simulink model "swingup_controller"  (R2015b)
settings: Solver=FixedStepDiscrete  StartTime=0.0  StopTime=tstop  FixedStep=T  RelTol=1e-3
values from neighbouring files (symbols this model uses):
  ABSALPHA_ON = 22.5 + (5)    (= 27.5)    [swingup_setup.m]
  Ad = ss_disc.A    [balance_setup.m]    (also in swingup_setup.m)
  alpha_cal = -(360/4096) * (pi/180)    (= -0.00153398078789)    [balance_setup.m]    (also in swingup_setup.m)
  ALPHAUR_ON = 60    [swingup_setup.m]
  Bd = ss_disc.B    [balance_setup.m]    (also in swingup_setup.m)
  bemf_lim = .25    (= 0.25)    [swingup_setup.m]
  Cd = ss_disc.C    [balance_setup.m]    (also in swingup_setup.m)
  Dd = ss_disc.D    [balance_setup.m]    (also in swingup_setup.m)
  Er = 0.42    [swingup_setup.m]
  eta_g = 0.9    [swingup_setup.m]
  eta_m = 0.69    [swingup_setup.m]
  g = 9.81    [swingup_setup.m]
  Jp = 0.0012    [swingup_setup.m]
  Kg = 70    [swingup_setup.m]
  km = 7.68e-3    (= 0.00768)    [swingup_setup.m]
  kt = 0.00768    [swingup_setup.m]
  Lp = 0.337    [swingup_setup.m]
  Lr = 0.216    [swingup_setup.m]
  Mp = 0.127    [swingup_setup.m]
  Mr = 0.257    [swingup_setup.m]
  mu = 5.5    [swingup_setup.m]
  Rm = 2.6    [swingup_setup.m]
  T = 0.001    [balance_setup.m]    (also in swingup_setup.m)
  theta_cal = -(360/4096) * (pi/180)    (= -0.00153398078789)    [balance_setup.m]    (also in swingup_setup.m)
  theta_HARDLIM = 160/180 * pi    (= 2.79252680319)    [swingup_setup.m]
  umax = 5    [swingup_setup.m]
  umax_LIM = tau/(Mr*Lr)    (= 11.565399581)    [swingup_setup.m]
  Vin_HARDLIM = 5    [swingup_setup.m]
undefined symbols (not defined in the file or in its folder): denV, Discrete, HIL, K_lqr, numV, Time
libraries: simulink x5, quarc_library x4, ctrlSharedLib x1
settings Model: SimulationMode=external  ExtModeTrigType=signal  ExtModeTrigDuration=200000  ExtModeTrigDirection=either  ExtModeTrigLevel=0.500000  Creator=shadar  LastModifiedBy=maxcrisafulli
settings SolverCC: PositivePriorityOrder=on
settings RTWCC: SystemTargetFile=quarc_win64.tlc  TemplateMakefile=quarc_default_tmf  Description=QUARC Win64 Target
settings STFCustomTargetCC: GeneratePreprocessorConditionals=Use local settings  CPPClassGenCompliant=off
settings GRTTargetCC: ParMdlRefBuildCompliant=off  CompOptLevelCompliant=off  CombineOutputUpdateFcns=off  MatFileLogging=off  CPPClassGenCompliant=off  GRTInterface=on  UseToolchainInfoCompliant=off  ExtMode=on  ExtModeMexFile=quarc_comm

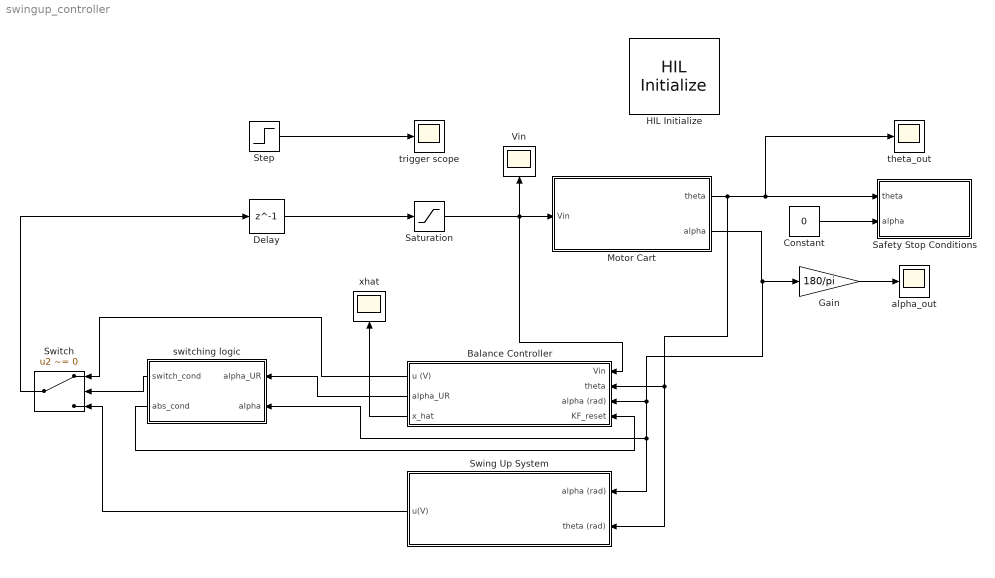
== system swingup_controller ==
  Balance Controller : Subsystem
  Constant : Constant  Value=0
  Delay : Delay  DelayLength=1  InitialCondition=0
  Gain : Gain  Gain=180/pi
  HIL Initialize : quarc_library/Data Acquisition/Generic/Configuration/HIL Initialize  object_name=HIL-1  board_type=q4  board_number=0  board_options=""  exclusive=off  active=on  hardware_clocks=[0:1]  clock_modes=[0 0]  initial_clock_frequencies=[]  set_clock_params_at_start=on  set_clock_params_at_switch_in=off  set_clock_frequencies_at_start=off  set_clock_frequencies_at_switch_in=off  analog_input_channels=[0:3]  analog_input_configurations=[]  analog_input_maximums=10  analog_input_minimums=-10  set_analog_input_params_at_start=off  set_analog_input_params_at_switch_in=off  analog_output_channels=[0:3]  analog_output_maximums=[10]  analog_output_minimums=[-10]  initial_analog_outputs=[0]  final_analog_outputs=[0]  watchdog_analog_outputs=0  set_analog_output_params_at_start=on  set_analog_output_params_at_switch_in=off  set_analog_outputs_at_start=on  set_analog_outputs_at_switch_in=off  set_analog_outputs_at_terminate=on  set_analog_outputs_at_switch_out=off  set_analog_outputs_on_watchdog=off  digital_input_channels=[]  digital_output_channels=[]  digital_output_configuration=[]  initial_digital_outputs=[1]  final_digital_outputs=[1]  watchdog_digital_outputs=[2]  set_digital_output_params_at_start=off  set_digital_output_params_at_switch_in=off  set_digital_outputs_at_start=on  set_digital_outputs_at_switch_in=off  set_digital_outputs_at_terminate=on  set_digital_outputs_at_switch_out=off  set_digital_outputs_on_watchdog=off  encoder_channels=[0:3]  quadrature=[4]  encoder_filter_frequency=(1/60e-9)/1  initial_encoder_counts=[0]  set_encoder_params_at_start=on  set_encoder_params_at_switch_in=off  set_encoder_counts_at_start=on  set_encoder_counts_at_switch_in=off  pwm_channels=[]  pwm_modes=[0]  pwm_frequency=(1/60e-9)/1024  pwm_configuration=[]  pwm_alignment=[]  pwm_polarity=[]  pwm_leading_deadband=[]  pwm_trailing_deadband=[]  initial_pwm_outputs=[0]  final_pwm_outputs=[0]  watchdog_pwm_outputs=[]  set_pwm_params_at_start=on  set_pwm_params_at_switch_in=off  set_pwm_outputs_at_start=on  set_pwm_outputs_at_switch_in=off  set_pwm_outputs_at_terminate=on  set_pwm_outputs_at_switch_out=off  set_pwm_outputs_on_watchdog=off  other_output_channels=[]  initial_other_outputs=[]  final_other_outputs=[]  watchdog_other_outputs=[]  set_other_outputs_at_start=off  set_other_outputs_at_switch_in=off  set_other_outputs_at_terminate=off  set_other_outputs_at_switch_out=off  set_other_outputs_on_watchdog=off
  "Motor Cart " : Subsystem
  Safety Stop Conditions : Subsystem
  Saturation : Saturate  UpperLimit=Vin_HARDLIM  LowerLimit=-Vin_HARDLIM
  Step : Step  Time=0.001  SampleTime=0
  Swing Up System : Subsystem
  Switch : Switch  Criteria=u2 ~= 0  Threshold=15/180 * pi
  Vin : Scope
  "alpha_out " : Scope
  switching logic : Subsystem
  theta_out : Scope
  trigger scope : Scope
  xhat : Scope
  wires:
  Step/1 -> trigger scope/1
  "Motor Cart "/1(theta) -> theta_out/1, Safety Stop Conditions/1(theta), Swing Up System/2(theta (rad)), Balance Controller/2(theta)
  "Motor Cart "/2(alpha) -> Swing Up System/1(alpha (rad)), switching logic/2(alpha), Balance Controller/3(alpha (rad)), Gain/1
  Saturation/1 -> Balance Controller/1(Vin), "Motor Cart "/1(Vin), Vin/1
  Delay/1 -> Saturation/1
  Constant/1 -> Safety Stop Conditions/2(alpha)
  Swing Up System/1(u(V)) -> Switch/3
  Switch/1 -> Delay/1
  Gain/1 -> "alpha_out "/1
  Balance Controller/3(x_hat) -> xhat/1
  Balance Controller/1(u (V)) -> Switch/1
  Balance Controller/2(alpha_UR) -> switching logic/1(alpha_UR)
  switching logic/1(switch_cond) -> Switch/2
  switching logic/2(abs_cond) -> Balance Controller/4("KF_reset ")

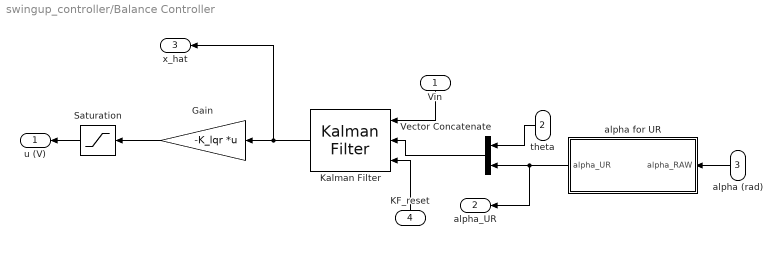
== system swingup_controller/Balance Controller ==
  Vin : Inport
  theta : Inport  Port=2
  alpha (rad) : Inport  Port=3
  "KF_reset " : Inport  Port=4
  Gain : Gain  Gain=-K_lqr  Multiplication=Matrix(K*u)
  Kalman Filter : ctrlSharedLib/Kalman Filter  TimeDomain=Discrete-Time  UseCurrentEstimator=on  ModelSource=Individual A, B, C, D matrices  ModelSourceVariable=ss(0.95,1,1,0,1)  A=Ad  B=Bd  C=Cd  D=Dd  NumberOfStates=1  NumberOfInputs=1  NumberOfOutputs=1  InitialEstimateSource=Dialog  X0=0  P0=10  UseK=off  UseGH=off  NumberOfProcessNoiseInputs=1  G=1  TimeInvariantG=on  H=0  TimeInvariantH=on  Q=1  TimeInvariantQ=on  R=300  TimeInvariantR=on  N=0  TimeInvariantN=on  AddInputPort=on  AddEnablePort=off  ExternalReset=Rising  OutputEstimatedY=off  OutputP=off  Ts=T
  Saturation : Saturate  UpperLimit=Vin_HARDLIM  LowerLimit=-Vin_HARDLIM
  Vector Concatenate : Concatenate
  alpha for UR : Subsystem
  u (V) : Outport
  alpha_UR : Outport  Port=2
  x_hat : Outport  Port=3
  wires:
  alpha for UR/1(alpha_UR) -> alpha_UR/1, Vector Concatenate/2
  theta/1 -> Vector Concatenate/1
  Vin/1 -> Kalman Filter/1
  Vector Concatenate/1 -> Kalman Filter/2
  alpha (rad)/1 -> alpha for UR/1(alpha_RAW)
  Gain/1 -> Saturation/1
  "KF_reset "/1 -> Kalman Filter/3
  Saturation/1 -> u (V)/1
  Kalman Filter/1 -> x_hat/1, Gain/1

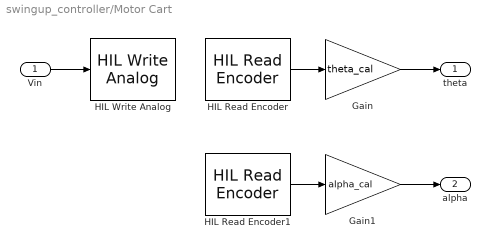
== system swingup_controller/Motor Cart  ==
  Vin : Inport
  Gain : Gain  Gain=theta_cal
  Gain1 : Gain  Gain=alpha_cal
  HIL Read Encoder : quarc_library/Data Acquisition/Generic/Immediate I//O/HIL Read Encoder  object_name=HIL-1  channels=0  sample_time=T  active=on  vector_output=on  data_type_mode=Inherit via back propagation  data_type=double
  HIL Read Encoder1 : quarc_library/Data Acquisition/Generic/Immediate I//O/HIL Read Encoder  object_name=HIL-1  channels=2  sample_time=qc_get_step_size  active=on  vector_output=off  data_type_mode=Inherit via back propagation  data_type=double
  HIL Write Analog : quarc_library/Data Acquisition/Generic/Immediate I//O/HIL Write Analog  object_name=HIL-1  channels=0  sample_time=T  active=off  vector_input=off
  theta : Outport
  alpha : Outport  Port=2
  wires:
  Vin/1 -> HIL Write Analog/1
  HIL Read Encoder/1 -> Gain/1
  Gain/1 -> theta/1
  HIL Read Encoder1/1 -> Gain1/1
  Gain1/1 -> alpha/1

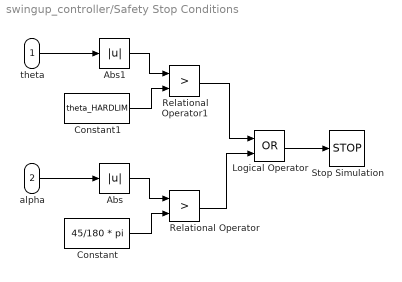
== system swingup_controller/Safety Stop Conditions ==
  theta : Inport
  alpha : Inport  Port=2
  Abs : Abs
  Abs1 : Abs
  Constant : Constant  Value=45/180 * pi
  Constant1 : Constant  Value=theta_HARDLIM
  Logical Operator : Logic  Operator=OR  AllPortsSameDT=off  OutDataTypeStr=boolean
  Relational Operator : RelationalOperator  Operator=>  OutDataTypeStr=boolean
  Relational Operator1 : RelationalOperator  Operator=>  OutDataTypeStr=boolean
  Stop Simulation : Stop
  wires:
  Abs/1 -> Relational Operator/1
  Constant/1 -> Relational Operator/2
  alpha/1 -> Abs/1
  theta/1 -> Abs1/1
  Relational Operator/1 -> Logical Operator/2
  Relational Operator1/1 -> Logical Operator/1
  Abs1/1 -> Relational Operator1/1
  Constant1/1 -> Relational Operator1/2
  Logical Operator/1 -> Stop Simulation/1

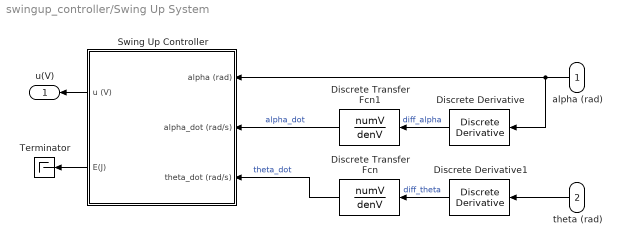
== system swingup_controller/Swing Up System ==
  alpha (rad) : Inport
  theta (rad) : Inport  Port=2
  Discrete Transfer Fcn : DiscreteTransferFcn  Numerator=numV  Denominator=denV
  Discrete Transfer Fcn1 : DiscreteTransferFcn  Numerator=numV  Denominator=denV
  Discrete Derivative : simulink/Discrete/Discrete Derivative  gainval=1.0  ICPrevScaledInput=0.0  InputProcessing=Inherited  OutMin=[]  OutMax=[]  OutDataType=fixdt(1, 16)  OutScaling=2^-10  DoSatur=off
  Discrete Derivative1 : simulink/Discrete/Discrete Derivative  gainval=1.0  ICPrevScaledInput=0.0  InputProcessing=Inherited  OutMin=[]  OutMax=[]  OutDataType=fixdt(1, 16)  OutScaling=2^-10  DoSatur=off
  Swing Up Controller : Subsystem
  Terminator : Terminator
  u(V) : Outport
  wires:
  theta (rad)/1 -> Discrete Derivative1/1
  Swing Up Controller/2(E(J)) -> Terminator/1
  alpha (rad)/1 -> Discrete Derivative/1, Swing Up Controller/1(alpha (rad))
  Discrete Transfer Fcn1/1 -> Swing Up Controller/2(alpha_dot (rad/s))  "alpha_dot"
  Discrete Derivative1/1 -> Discrete Transfer Fcn/1  "diff_theta"
  Discrete Transfer Fcn/1 -> Swing Up Controller/3(theta_dot (rad/s))  "theta_dot"
  Discrete Derivative/1 -> Discrete Transfer Fcn1/1  "diff_alpha"
  Swing Up Controller/1(u (V)) -> u(V)/1

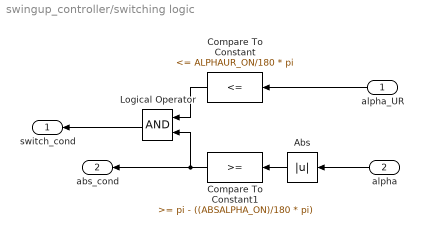
== system swingup_controller/switching logic ==
  alpha_UR : Inport
  alpha : Inport  Port=2
  Abs : Abs
  Compare To Constant : simulink/Logic and Bit Operations/Compare To Constant  relop=<=  const=ALPHAUR_ON/180 * pi  OutDataTypeStr=boolean
  Compare To Constant1 : simulink/Logic and Bit Operations/Compare To Constant  relop=>=  const=pi - ((ABSALPHA_ON)/180 * pi)  OutDataTypeStr=boolean
  Logical Operator : Logic  AllPortsSameDT=off  OutDataTypeStr=boolean
  switch_cond : Outport
  abs_cond : Outport  Port=2
  wires:
  Compare To Constant1/1 -> abs_cond/1, Logical Operator/2
  Logical Operator/1 -> switch_cond/1
  alpha_UR/1 -> Compare To Constant/1
  Abs/1 -> Compare To Constant1/1
  Compare To Constant/1 -> Logical Operator/1
  alpha/1 -> Abs/1

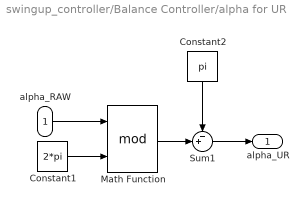
== system swingup_controller/Balance Controller/alpha for UR ==
  alpha_RAW : Inport
  Constant1 : Constant  Value=2*pi
  Constant2 : Constant  Value=pi
  Math Function : Math  Operator=mod  SaturateOnIntegerOverflow=on
  Sum1 : Sum  Inputs=-+|
  alpha_UR : Outport
  wires:
  Constant1/1 -> Math Function/2
  Math Function/1 -> Sum1/2
  Sum1/1 -> alpha_UR/1
  alpha_RAW/1 -> Math Function/1
  Constant2/1 -> Sum1/1

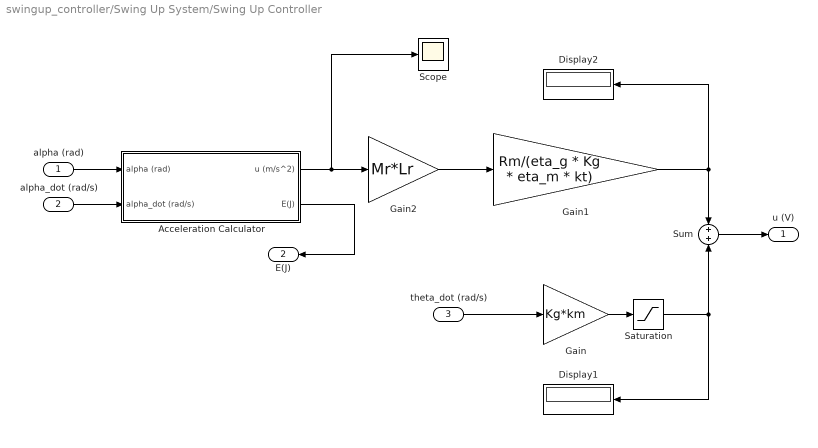
== system swingup_controller/Swing Up System/Swing Up Controller ==
  alpha (rad) : Inport
  alpha_dot (rad/s) : Inport  Port=2
  theta_dot (rad/s) : Inport  Port=3
  Acceleration Calculator : Subsystem
  Display1 : Display
  Display2 : Display
  Gain : Gain  Gain=Kg*km
  Gain1 : Gain  Gain=Rm/(eta_g * Kg * eta_m * kt)
  Gain2 : Gain  Gain=Mr*Lr
  Saturation : Saturate  UpperLimit=bemf_lim  LowerLimit=-bemf_lim
  Scope : Scope
  Sum : Sum  Inputs=+|+
  u (V) : Outport
  E(J) : Outport  Port=2
  wires:
  alpha (rad)/1 -> Acceleration Calculator/1(alpha (rad))
  Acceleration Calculator/2(E(J)) -> E(J)/1
  theta_dot (rad/s)/1 -> Gain/1
  Sum/1 -> u (V)/1
  Gain/1 -> Saturation/1
  Acceleration Calculator/1(u (m/s^2)) -> Scope/1, Gain2/1
  Gain2/1 -> Gain1/1
  Gain1/1 -> Display2/1, Sum/1
  Saturation/1 -> Sum/2, Display1/1
  alpha_dot (rad/s)/1 -> Acceleration Calculator/2(alpha_dot (rad/s))

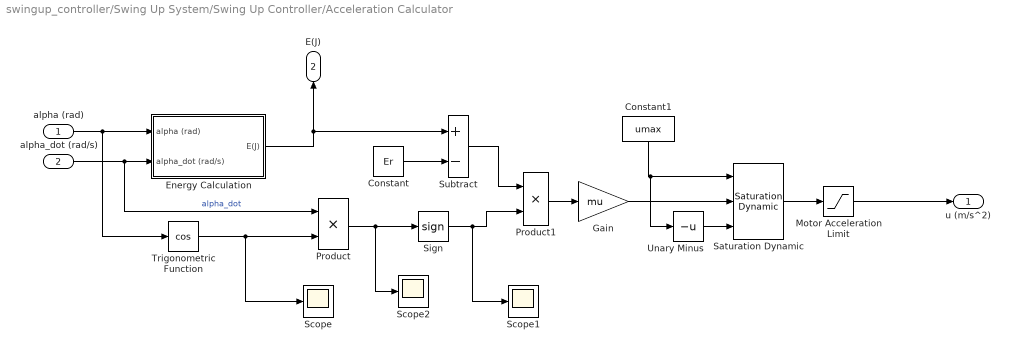
== system swingup_controller/Swing Up System/Swing Up Controller/Acceleration Calculator ==
  alpha (rad) : Inport
  alpha_dot (rad/s) : Inport  Port=2
  Constant : Constant  Value=Er
  Constant1 : Constant  Value=umax
  Energy Calculation : Subsystem
  Gain : Gain  Gain=mu
  Motor Acceleration Limit : Saturate  UpperLimit=umax_LIM  LowerLimit=-umax_LIM
  Product : Product
  Product1 : Product
  Saturation Dynamic : simulink/Discontinuities/Saturation Dynamic  OutMin=[]  OutMax=[]  OutDataTypeStr=Inherit: Same as second input  OutDataType=fixdt(1, 16)  OutScaling=2^-10  DoSatur=off
  Scope : Scope
  Scope1 : Scope
  Scope2 : Scope
  Sign : Signum
  Subtract : Sum  Inputs=+-
  Trigonometric Function : Trigonometry  Operator=cos
  Unary Minus : UnaryMinus
  u (m/s^2) : Outport
  E(J) : Outport  Port=2
  wires:
  alpha (rad)/1 -> Trigonometric Function/1, Energy Calculation/1(alpha (rad))
  Energy Calculation/1(E(J)) -> E(J)/1, Subtract/1
  alpha_dot (rad/s)/1 -> Product/1, Energy Calculation/2(alpha_dot (rad/s))  "alpha_dot"
  Trigonometric Function/1 -> Scope/1, Product/2
  Product/1 -> Scope2/1, Sign/1
  Constant/1 -> Subtract/2
  Subtract/1 -> Product1/1
  Sign/1 -> Scope1/1, Product1/2
  Product1/1 -> Gain/1
  Gain/1 -> Saturation Dynamic/2
  Unary Minus/1 -> Saturation Dynamic/3
  Constant1/1 -> Saturation Dynamic/1, Unary Minus/1
  Saturation Dynamic/1 -> Motor Acceleration Limit/1
  Motor Acceleration Limit/1 -> u (m/s^2)/1

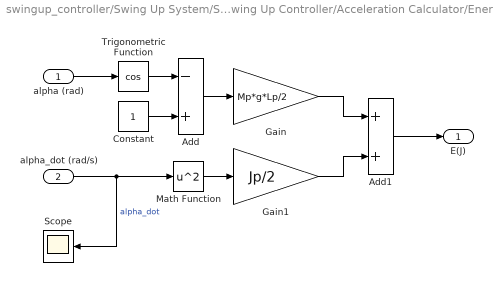
== system swingup_controller/Swing Up System/Swing Up Controller/Acceleration Calculator/Energy Calculation ==
  alpha (rad) : Inport
  alpha_dot (rad/s) : Inport  Port=2
  Add : Sum  Inputs=-+
  Add1 : Sum
  Constant : Constant
  Gain : Gain  Gain=Mp*g*Lp/2
  Gain1 : Gain  Gain=Jp/2
  Math Function : Math  Operator=square  SaturateOnIntegerOverflow=on
  Scope : Scope
  Trigonometric Function : Trigonometry  Operator=cos  ApproximationMethod=CORDIC
  E(J) : Outport
  wires:
  alpha (rad)/1 -> Trigonometric Function/1
  Trigonometric Function/1 -> Add/1
  Constant/1 -> Add/2
  Add/1 -> Gain/1
  alpha_dot (rad/s)/1 -> Scope/1, Math Function/1  "alpha_dot"
  Math Function/1 -> Gain1/1
  Gain1/1 -> Add1/2
  Gain/1 -> Add1/1
  Add1/1 -> E(J)/1
